simulink model "relay_3_vi_tri_r2015a"  (R2016b)
settings: Solver=ode4  StartTime=0.0  StopTime=100  FixedStep=0.001  RelTol=1e-3
settings Model: Creator=ryell  LastModifiedBy=ADMIN
settings OptimizationCC: LifeSpan=inf
settings DebuggingCC: SFExecutionAtInitializationDiag=none
settings HardwareCC: ProdBitPerSizeT=32  ProdBitPerPtrDiffT=32  ProdWordSize=32  ProdHWDeviceType=Specified

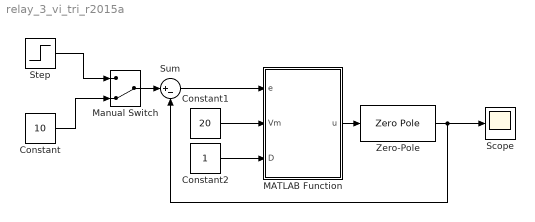
== system relay_3_vi_tri_r2015a ==
  Constant : Constant  Value=10
  Constant1 : Constant  Value=20
  Constant2 : Constant
  MATLAB Function : MATLAB Function  TreatAsAtomicUnit=on
  Manual Switch : ManualSwitch  CurrentSetting=0
  Scope : Scope
  Step : Step  Time=2  Before=10  After=0  SampleTime=0
  Sum : Sum  Inputs=|+-
  Zero-Pole : ZeroPole  Zeros=[]  Poles=[-1 -1 -1]
  wires:
  Zero-Pole/1 -> Scope/1, Sum/2
  Sum/1 -> MATLAB Function/1(e)
  MATLAB Function/1(u) -> Zero-Pole/1
  Manual Switch/1 -> Sum/1
  Step/1 -> Manual Switch/1
  Constant/1 -> Manual Switch/2
  Constant2/1 -> MATLAB Function/3(D)
  Constant1/1 -> MATLAB Function/2(Vm)

== matlab function relay_3_vi_tri_r2015a/MATLAB Function ==
  data: e input; u output; Vm input; D input
function u = relay3(e,Vm,D)
if (e < -D)
    u = -Vm;
elseif (e < D)
    u = 0;
else
    u = Vm;
end
end
